simulink model "BRAM_STN_32bit"  (R2021a)
settings: Solver=VariableStepAuto  StartTime=0.0  StopTime=7500.0  RelTol=1e-3
values from neighbouring files (symbols this model uses):
  F_bit = 27    [main.m]
undefined symbols (not defined in the file or in its folder): S, vsva2197, xcvc1902
libraries: xbsIndex_r4 x99, ModelComposer x25, simulink x1
settings Model: Creator=maruf  LastModifiedBy=maruf

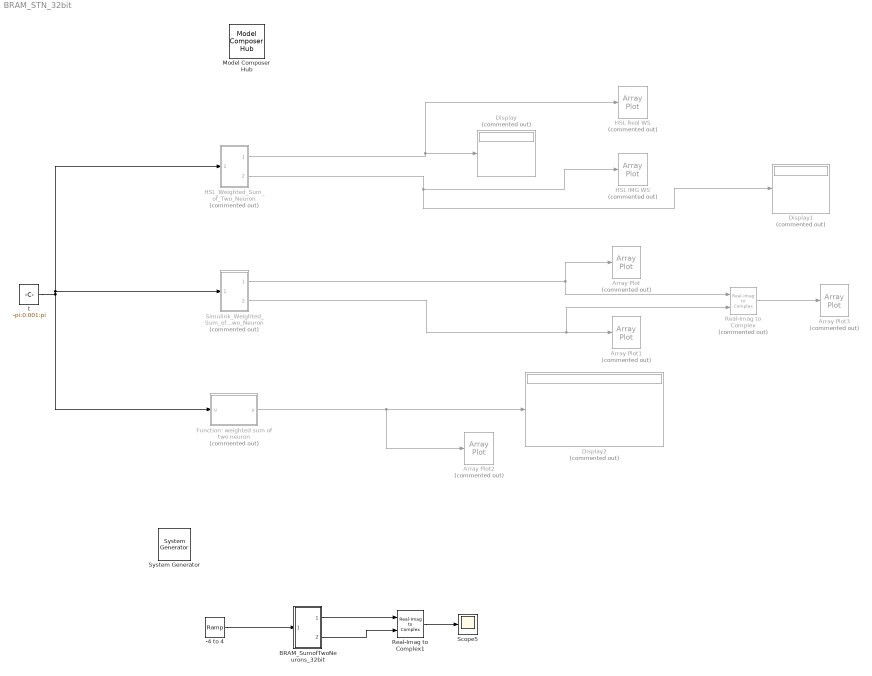
== system BRAM_STN_32bit ==
  " System Generator" : xbsIndex_r4/ System Generator  Tag=genX  xilinxfamily=zynq  part=xc7z020  speed=-1  package=clg484  synthesis_tool=Vivado  clock_wrapper=Clock Enables  directory=E:/FPGAProject/01102022/FPGAResearch/5_Final_Submission/Simulink/BRAM_LT_Based/BRAM32bit/gen_withRegister  proj_type=Vivado  Synth_file=Vivado Synthesis Defaults  Impl_file=Vivado Implementation Defaults  testbench=off  simulink_period=1  sysclk_period=100  dcm_input_clock_period=10  incr_netlist=off  trim_vbits=Everywhere in SubSystem  dbl_ovrd=According to Block Masks  core_generation=According to Block Masks  run_coregen=off  deprecated_control=off  eval_field=0  block_type=sysgen
  -4 to 4 : simulink/Sources/Ramp  slope=1/1000  start=0  InitialOutput=-4
  Array Plot : ArrayPlot  Commented=on  WindowPosition=[5.000000,516.000000,510.000000,316.000000,]  YLimits=[-0.9622504313624441,0.9622504139961428]  DefaultConfigurationName=dsp.scopes.ArrayPlotBlockSpecification
  Array Plot1 : ArrayPlot  Commented=on  WindowPosition=[-2.000000,147.000000,512.000000,337.000000,]  YLimits=[-1.2499999481465376,1.24999953331884]  DefaultConfigurationName=dsp.scopes.ArrayPlotBlockSpecification
  Array Plot2 : ArrayPlot  Commented=on  WindowPosition=[2.000000,179.000000,518.000000,354.000000,]  YLimits=[-1.249996371900796,1.2499673471071675]  ShowLegend=on  DefaultConfigurationName=dsp.scopes.ArrayPlotBlockSpecification
  Array Plot3 : ArrayPlot  Commented=on  WindowPosition=[525.000000,102.000000,526.000000,333.000000,]  YLimits=[-1.249993408699066,1.2499406782915958]  ShowLegend=on  DefaultConfigurationName=dsp.scopes.ArrayPlotBlockSpecification
  BRAM_SumofTwoNeurons_32bit : Subsystem
  Display : Display  Commented=on
  Display1 : Display  Commented=on
  Display2 : Display  Commented=on
  Function: weighted sum of two neuron : MATLAB Function  Commented=on  TreatAsAtomicUnit=on
  HSL IMG WS : ArrayPlot  Commented=on  WindowPosition=[651.000000,15.000000,537.000000,382.000000,]  YLimits=[-1.2499999481465376,1.24999953331884]  DefaultConfigurationName=dsp.scopes.ArrayPlotBlockSpecification
  HSL Real WS : ArrayPlot  Commented=on  WindowPosition=[999.000000,483.000000,539.000000,349.000000,]  YLimits=[-0.9622504313624441,0.9622504139961428]  DefaultConfigurationName=dsp.scopes.ArrayPlotBlockSpecification
  HSL_Weighted_Sum_of_Two_Neuron : Subsystem  Commented=on
  Model Composer Hub : ModelComposer/Model Composer Hub  CodeGeneration=off  SubsystemName=HSL_Weighted_Sum_of_Two_Neuron  TargetDirectory=E:/FPGAProject/01102022/FPGAResearch/25102022_MC/twoNeuron/simulink/code  ExportType=System Generator  IpVendor=xilinx.com  IpLibrary=hls  IpVersion=1.0  IpHWLanguage=Verilog  AieCompilerOptions={}  CreateTestbench=off  TestbenchStackSize=10  RunAieSim=off  AieSimTimeout=50000  RunAieSimProfiling=off  LaunchVitisAnalyzer=off  PlotOutput=off  RunX86Sim=off  X86SimTimeout=10  PlatformType=Not Specified  ProjDevice=xcvc1902-vsva2197-2MP-e-S  ProjDevicePart=xcvc1902-vsva2197-2MP-e-S  SamplePeriod=-1  ClockFrequency=200  DataPathParallelism=1
  Real-Imag to Complex : ModelComposer/Real-Imag to Complex  Commented=on  Input=Real and imag  ConstantPart=0
  Real-Imag to Complex1 : ModelComposer/Real-Imag to Complex  Input=Real and imag  ConstantPart=0
  Scope5 : Scope
  Simulink_Weighted_Sum_of_Two_Neuron : Subsystem  Commented=on
  t : Constant  Value=-pi:0.001:pi
  wires:
  t/1 -> Simulink_Weighted_Sum_of_Two_Neuron/1(In1), HSL_Weighted_Sum_of_Two_Neuron/1(In1), Function: weighted sum of two neuron/1(u)
  Function: weighted sum of two neuron/1(y) -> Array Plot2/1, Display2/1
  Simulink_Weighted_Sum_of_Two_Neuron/1(Out1) -> Array Plot/1, Real-Imag to Complex/1
  Simulink_Weighted_Sum_of_Two_Neuron/2(Out2) -> Real-Imag to Complex/2, Array Plot1/1
  HSL_Weighted_Sum_of_Two_Neuron/1(Out1) -> HSL Real WS/1, Display/1
  HSL_Weighted_Sum_of_Two_Neuron/2(Out2) -> Display1/1, HSL IMG WS/1
  Real-Imag to Complex/1 -> Array Plot3/1
  Real-Imag to Complex1/1 -> Scope5/1
  -4 to 4/1 -> BRAM_SumofTwoNeurons_32bit/1(Input)
  BRAM_SumofTwoNeurons_32bit/1(Out1) -> Real-Imag to Complex1/1
  BRAM_SumofTwoNeurons_32bit/2(Out2) -> Real-Imag to Complex1/2

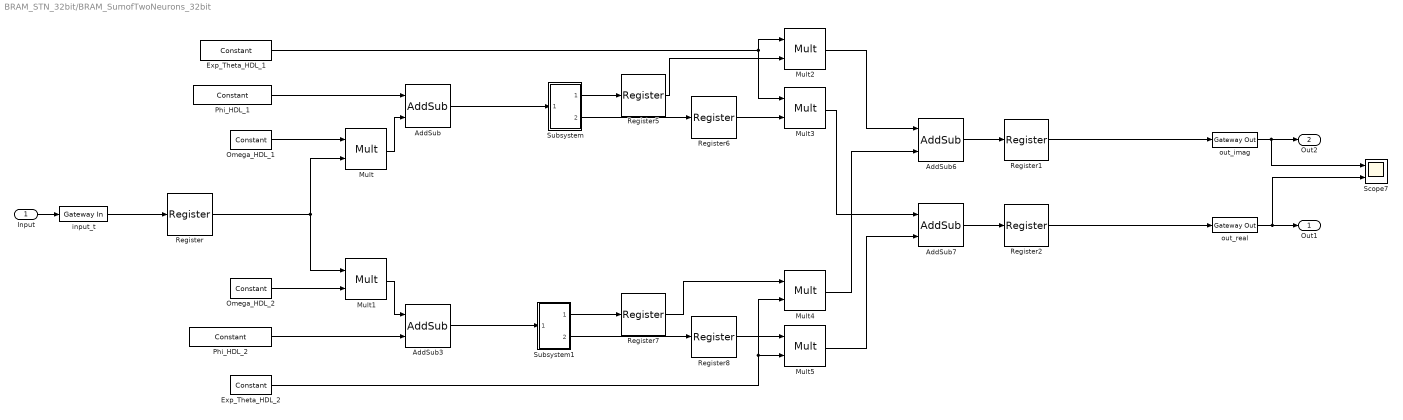
== system BRAM_STN_32bit/BRAM_SumofTwoNeurons_32bit ==
  Input : Inport
  AddSub{,3,6..7} (4 alike) : xbsIndex_r4/AddSub  mode=Addition  use_carryin=off  use_carryout=off  en=off  latency=1  precision=User Defined  arith_type="Signed  (2's comp)"  n_bits=N_bit  bin_pt=F_bit  quantization=Truncate  overflow=Wrap  use_behavioral_HDL=off  hw_selection=Fabric  pipelined=off  dbl_ovrd=off  block_type=addsub
  Exp_Theta_HDL_1 : xbsIndex_r4/Constant  const=2  gui_display_data_type=Fixed-point  arith_type=Signed (2's comp)  n_bits=N_bit  bin_pt=F_bit  preci_type=Single  exp_width=8  frac_width=24  explicit_period=on  period=1  equ=P=C  opselect=C  inp2=PCIN>>17  opr=+  inp1=P  carry=CIN  dbl_ovrd=off  block_type=constant
  Exp_Theta_HDL_2 : xbsIndex_r4/Constant  const=2  gui_display_data_type=Fixed-point  arith_type=Signed (2's comp)  n_bits=N_bit  bin_pt=F_bit  preci_type=Single  exp_width=8  frac_width=24  explicit_period=on  period=1  equ=P=C  opselect=C  inp2=PCIN>>17  opr=+  inp1=P  carry=CIN  dbl_ovrd=off  block_type=constant
  Mult{,1..5} (6 alike) : xbsIndex_r4/Mult  precision=User Defined  arith_type="Signed  (2's comp)"  n_bits=N_bit  bin_pt=F_bit  quantization=Truncate  overflow=Wrap  en=off  latency=3  use_behavioral_HDL=off  opt=Speed  use_embedded=on  optimum_pipeline=off  pipeline=on  dbl_ovrd=off  use_rpm=on  placement_style=Triangular  block_type=mult
  Omega_HDL_1 : xbsIndex_r4/Constant  const=1  gui_display_data_type=Fixed-point  arith_type=Signed (2's comp)  n_bits=N_bit  bin_pt=F_bit  preci_type=Single  exp_width=8  frac_width=24  explicit_period=on  period=1  equ=P=C  opselect=C  inp2=PCIN>>17  opr=+  inp1=P  carry=CIN  dbl_ovrd=off  block_type=constant
  Omega_HDL_2 : xbsIndex_r4/Constant  const=2  gui_display_data_type=Fixed-point  arith_type=Signed (2's comp)  n_bits=N_bit  bin_pt=F_bit  preci_type=Single  exp_width=8  frac_width=24  explicit_period=on  period=1  equ=P=C  opselect=C  inp2=PCIN>>17  opr=+  inp1=P  carry=CIN  dbl_ovrd=off  block_type=constant
  Phi_HDL_1 : xbsIndex_r4/Constant  const=3.14/2  gui_display_data_type=Fixed-point  arith_type=Signed (2's comp)  n_bits=N_bit  bin_pt=F_bit  preci_type=Single  exp_width=8  frac_width=24  explicit_period=on  period=1  equ=P=C  opselect=C  inp2=PCIN>>17  opr=+  inp1=P  carry=CIN  dbl_ovrd=off  block_type=constant
  Phi_HDL_2 : xbsIndex_r4/Constant  const=3.14/2  gui_display_data_type=Fixed-point  arith_type=Signed (2's comp)  n_bits=N_bit  bin_pt=F_bit  preci_type=Single  exp_width=8  frac_width=24  explicit_period=on  period=1  equ=P=C  opselect=C  inp2=PCIN>>17  opr=+  inp1=P  carry=CIN  dbl_ovrd=off  block_type=constant
  Register{,1..2,5..8} (7 alike) : xbsIndex_r4/Register  init=0  rst=off  en=off  dbl_ovrd=off  block_type=register
  Scope7 : Scope  NumInputPorts=2
  Subsystem : Subsystem
  Subsystem1 : Subsystem
  input_t : xbsIndex_r4/Gateway In  gui_display_data_type=Fixed-point  arith_type="Signed  (2's comp)"  n_bits=N_bit  bin_pt=F_bit  preci_type=Single  exp_width=8  frac_width=24  rows=1  columns=1  quantization=Truncate  overflow=Wrap  period=1  UseAsADC=off  ADCChannel='1'  interface=None  automatic_assignment=on  address_offset=hex2dec('00')  intf_name=''  intf_description=''  default_value=0  timing_constraint=None  locs_specified=off  LOCs={}  io_standard={}  inherit_from_input=off  hdl_port=on  dbl_ovrd=off  block_type=gatewayin
  out_imag : xbsIndex_r4/Gateway Out  inherit_from_input=off  hdl_port=on  rows=1  columns=1  UseAsDAC=off  DACChannel='1'  interface=None  automatic_assignment=on  address_offset=hex2dec('00')  intf_name=''  intf_description=''  timing_constraint=None  locs_specified=off  LOCs={}  io_standard={}  block_type=gatewayout
  out_real : xbsIndex_r4/Gateway Out  inherit_from_input=off  hdl_port=on  rows=1  columns=1  UseAsDAC=off  DACChannel='1'  interface=None  automatic_assignment=on  address_offset=hex2dec('00')  intf_name=''  intf_description=''  timing_constraint=None  locs_specified=off  LOCs={}  io_standard={}  block_type=gatewayout
  Out1 : Outport
  Out2 : Outport  Port=2
  wires:
  AddSub/1 -> Subsystem/1(In1)
  Phi_HDL_1/1 -> AddSub/1
  Mult/1 -> AddSub/2
  Omega_HDL_1/1 -> Mult/1
  Exp_Theta_HDL_1/1 -> Mult2/1, Mult3/1
  Omega_HDL_2/1 -> Mult1/2
  Mult1/1 -> AddSub3/1
  Phi_HDL_2/1 -> AddSub3/2
  Exp_Theta_HDL_2/1 -> Mult5/2, Mult4/2
  Mult2/1 -> AddSub6/1
  Mult4/1 -> AddSub6/2
  Mult3/1 -> AddSub7/1
  Mult5/1 -> AddSub7/2
  out_imag/1 -> Out2/1, Scope7/1
  AddSub7/1 -> Register2/1
  out_real/1 -> Scope7/2, Out1/1
  Input/1 -> input_t/1
  input_t/1 -> Register/1
  AddSub6/1 -> Register1/1
  Subsystem/1(Out1) -> Register5/1
  Subsystem/2(Out2) -> Register6/1
  AddSub3/1 -> Subsystem1/1(In1)
  Subsystem1/2(Out2) -> Register8/1
  Subsystem1/1(Out1) -> Register7/1
  Register/1 -> Mult/2, Mult1/1
  Register1/1 -> out_imag/1
  Register2/1 -> out_real/1
  Register5/1 -> Mult2/2
  Register6/1 -> Mult3/2
  Register7/1 -> Mult4/1
  Register8/1 -> Mult5/1

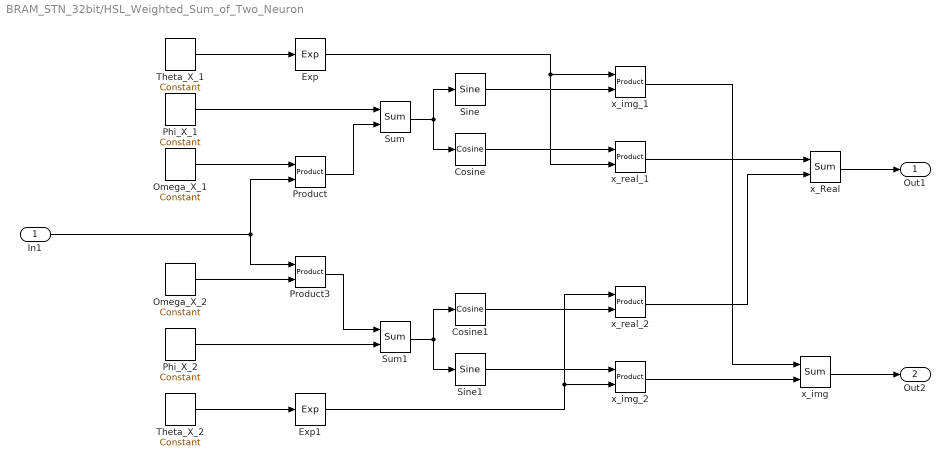
== system BRAM_STN_32bit/HSL_Weighted_Sum_of_Two_Neuron ==
  In1 : Inport
  Cosine : ModelComposer/Cosine
  Cosine1 : ModelComposer/Cosine
  Exp : ModelComposer/Exp
  Exp1 : ModelComposer/Exp
  Omega_X_1 : ModelComposer/Constant  Value=1  VectorParams1D=off  SampleTime=inf  OutDataType=double  TypeExp=''  Signedness=Signed  WordLength=16  FractionalLength=0  RoundingMode=Truncation to minus infinity  OverflowMode=Wrap around
  Omega_X_2 : ModelComposer/Constant  Value=3  SampleTime=inf  OutDataType=double  TypeExp=''  Signedness=Signed  WordLength=16  FractionalLength=0  RoundingMode=Truncation to minus infinity  OverflowMode=Wrap around
  Phi_X_1 : ModelComposer/Constant  Value=pi/2  SampleTime=inf  OutDataType=double  TypeExp=''  Signedness=Signed  WordLength=16  FractionalLength=0  RoundingMode=Truncation to minus infinity  OverflowMode=Wrap around
  Phi_X_2 : ModelComposer/Constant  Value=pi/2  SampleTime=inf  OutDataType=double  TypeExp=''  Signedness=Signed  WordLength=16  FractionalLength=0  RoundingMode=Truncation to minus infinity  OverflowMode=Wrap around
  Product : ModelComposer/Product
  Product3 : ModelComposer/Product
  Sine : ModelComposer/Sine
  Sine1 : ModelComposer/Sine
  Sum : ModelComposer/Sum
  Sum1 : ModelComposer/Sum
  Theta_X_1 : ModelComposer/Constant  Value=log(0.5)  SampleTime=inf  OutDataType=double  TypeExp=''  Signedness=Signed  WordLength=16  FractionalLength=0  RoundingMode=Truncation to minus infinity  OverflowMode=Wrap around
  Theta_X_2 : ModelComposer/Constant  Value=log(0.5)  SampleTime=inf  OutDataType=double  TypeExp=''  Signedness=Signed  WordLength=16  FractionalLength=0  RoundingMode=Truncation to minus infinity  OverflowMode=Wrap around
  x_Real : ModelComposer/Sum
  x_img : ModelComposer/Sum
  x_img_1 : ModelComposer/Product
  x_img_2 : ModelComposer/Product
  x_real_1 : ModelComposer/Product
  x_real_2 : ModelComposer/Product
  Out1 : Outport
  Out2 : Outport  Port=2
  wires:
  Product/1 -> Sum/2
  Cosine/1 -> x_real_1/1
  Sum/1 -> Sine/1, Cosine/1
  Exp/1 -> x_real_1/2, x_img_1/1
  Sine/1 -> x_img_1/2
  In1/1 -> Product/2, Product3/1
  Phi_X_1/1 -> Sum/1
  Omega_X_1/1 -> Product/1
  Omega_X_2/1 -> Product3/2
  Phi_X_2/1 -> Sum1/2
  Product3/1 -> Sum1/1
  Sum1/1 -> Cosine1/1, Sine1/1
  Theta_X_2/1 -> Exp1/1
  Exp1/1 -> x_real_2/1, x_img_2/2
  Sine1/1 -> x_img_2/1
  Cosine1/1 -> x_real_2/2
  x_img/1 -> Out2/1
  x_Real/1 -> Out1/1
  x_real_2/1 -> x_Real/2
  x_real_1/1 -> x_Real/1
  x_img_2/1 -> x_img/2
  x_img_1/1 -> x_img/1
  Theta_X_1/1 -> Exp/1

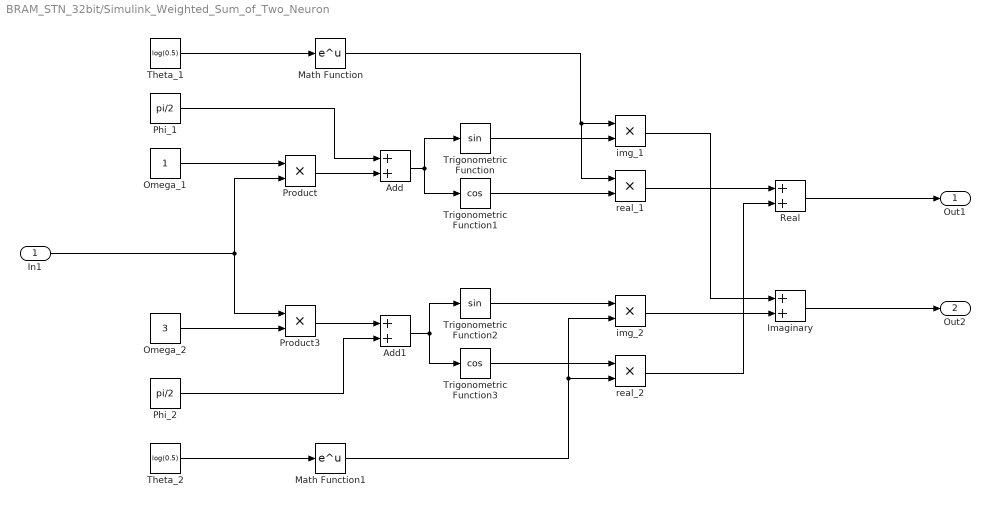
== system BRAM_STN_32bit/Simulink_Weighted_Sum_of_Two_Neuron ==
  In1 : Inport
  Add : Sum
  Add1 : Sum
  Imaginary : Sum
  Math Function : Math  SaturateOnIntegerOverflow=on
  Math Function1 : Math  SaturateOnIntegerOverflow=on
  Omega_1 : Constant
  Omega_2 : Constant  Value=3
  Phi_1 : Constant  Value=pi/2
  Phi_2 : Constant  Value=pi/2
  Product : Product
  Product3 : Product
  Real : Sum
  Theta_1 : Constant  Value=log(0.5)
  Theta_2 : Constant  Value=log(0.5)
  Trigonometric Function : Trigonometry
  Trigonometric Function1 : Trigonometry  Operator=cos
  Trigonometric Function2 : Trigonometry
  Trigonometric Function3 : Trigonometry  Operator=cos
  img_1 : Product
  img_2 : Product
  real_1 : Product
  real_2 : Product
  Out1 : Outport
  Out2 : Outport  Port=2
  wires:
  Theta_2/1 -> Math Function1/1
  Trigonometric Function1/1 -> real_1/2
  real_1/1 -> Real/1
  real_2/1 -> Real/2
  Add/1 -> Trigonometric Function1/1, Trigonometric Function/1
  Omega_1/1 -> Product/1
  Trigonometric Function3/1 -> real_2/1
  Omega_2/1 -> Product3/2
  img_2/1 -> Imaginary/2
  Math Function/1 -> real_1/1, img_1/1
  Trigonometric Function2/1 -> img_2/1
  Theta_1/1 -> Math Function/1
  In1/1 -> Product/2, Product3/1
  Product3/1 -> Add1/1
  Product/1 -> Add/2
  img_1/1 -> Imaginary/1
  Trigonometric Function/1 -> img_1/2
  Math Function1/1 -> img_2/2, real_2/2
  Phi_1/1 -> Add/1
  Add1/1 -> Trigonometric Function2/1, Trigonometric Function3/1
  Real/1 -> Out1/1
  Phi_2/1 -> Add1/2
  Imaginary/1 -> Out2/1

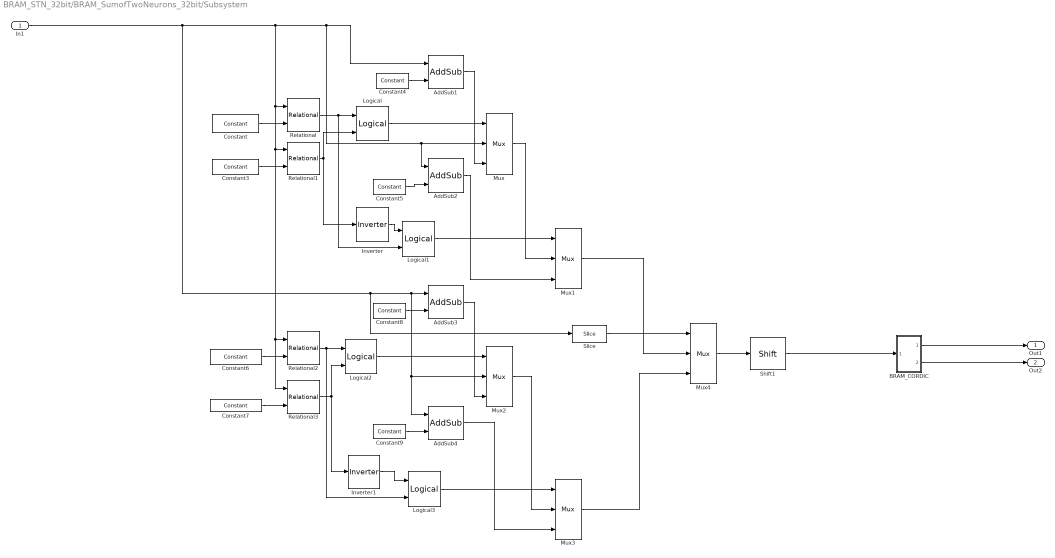
== system BRAM_STN_32bit/BRAM_SumofTwoNeurons_32bit/Subsystem ==
  In1 : Inport
  AddSub1 : xbsIndex_r4/AddSub  mode=Subtraction  use_carryin=off  use_carryout=off  en=off  latency=1  precision=User Defined  arith_type="Signed  (2's comp)"  n_bits=N_bit  bin_pt=F_bit  quantization=Truncate  overflow=Wrap  use_behavioral_HDL=off  hw_selection=Fabric  pipelined=off  dbl_ovrd=off  block_type=addsub
  AddSub2 : xbsIndex_r4/AddSub  mode=Subtraction  use_carryin=off  use_carryout=off  en=off  latency=1  precision=User Defined  arith_type="Signed  (2's comp)"  n_bits=N_bit  bin_pt=F_bit  quantization=Truncate  overflow=Wrap  use_behavioral_HDL=off  hw_selection=Fabric  pipelined=off  dbl_ovrd=off  block_type=addsub
  AddSub3 : xbsIndex_r4/AddSub  mode=Addition  use_carryin=off  use_carryout=off  en=off  latency=1  precision=User Defined  arith_type="Signed  (2's comp)"  n_bits=N_bit  bin_pt=F_bit  quantization=Truncate  overflow=Wrap  use_behavioral_HDL=off  hw_selection=Fabric  pipelined=off  dbl_ovrd=off  block_type=addsub
  AddSub4 : xbsIndex_r4/AddSub  mode=Addition  use_carryin=off  use_carryout=off  en=off  latency=1  precision=User Defined  arith_type="Signed  (2's comp)"  n_bits=N_bit  bin_pt=F_bit  quantization=Truncate  overflow=Wrap  use_behavioral_HDL=off  hw_selection=Fabric  pipelined=off  dbl_ovrd=off  block_type=addsub
  BRAM_CORDIC : Subsystem
  Constant : xbsIndex_r4/Constant  const=3.14  gui_display_data_type=Fixed-point  arith_type=Signed (2's comp)  n_bits=N_bit  bin_pt=F_bit  preci_type=Single  exp_width=8  frac_width=24  explicit_period=on  period=1  equ=P=C  opselect=C  inp2=PCIN>>17  opr=+  inp1=P  carry=CIN  dbl_ovrd=off  block_type=constant
  Constant3 : xbsIndex_r4/Constant  const=9.42  gui_display_data_type=Fixed-point  arith_type=Signed (2's comp)  n_bits=N_bit  bin_pt=F_bit  preci_type=Single  exp_width=8  frac_width=24  explicit_period=on  period=1  equ=P=C  opselect=C  inp2=PCIN>>17  opr=+  inp1=P  carry=CIN  dbl_ovrd=off  block_type=constant
  Constant4 : xbsIndex_r4/Constant  const=6.28  gui_display_data_type=Fixed-point  arith_type=Signed (2's comp)  n_bits=N_bit  bin_pt=F_bit  preci_type=Single  exp_width=8  frac_width=24  explicit_period=on  period=1  equ=P=C  opselect=C  inp2=PCIN>>17  opr=+  inp1=P  carry=CIN  dbl_ovrd=off  block_type=constant
  Constant5 : xbsIndex_r4/Constant  const=12.56  gui_display_data_type=Fixed-point  arith_type=Signed (2's comp)  n_bits=N_bit  bin_pt=F_bit  preci_type=Single  exp_width=8  frac_width=24  explicit_period=on  period=1  equ=P=C  opselect=C  inp2=PCIN>>17  opr=+  inp1=P  carry=CIN  dbl_ovrd=off  block_type=constant
  Constant6 : xbsIndex_r4/Constant  const=-3.14  gui_display_data_type=Fixed-point  arith_type=Signed (2's comp)  n_bits=N_bit  bin_pt=F_bit  preci_type=Single  exp_width=8  frac_width=24  explicit_period=on  period=1  equ=P=C  opselect=C  inp2=PCIN>>17  opr=+  inp1=P  carry=CIN  dbl_ovrd=off  block_type=constant
  Constant7 : xbsIndex_r4/Constant  const=-9.42  gui_display_data_type=Fixed-point  arith_type=Signed (2's comp)  n_bits=N_bit  bin_pt=F_bit  preci_type=Single  exp_width=8  frac_width=24  explicit_period=on  period=1  equ=P=C  opselect=C  inp2=PCIN>>17  opr=+  inp1=P  carry=CIN  dbl_ovrd=off  block_type=constant
  Constant8 : xbsIndex_r4/Constant  const=6.28  gui_display_data_type=Fixed-point  arith_type=Signed (2's comp)  n_bits=N_bit  bin_pt=F_bit  preci_type=Single  exp_width=8  frac_width=24  explicit_period=on  period=1  equ=P=C  opselect=C  inp2=PCIN>>17  opr=+  inp1=P  carry=CIN  dbl_ovrd=off  block_type=constant
  Constant9 : xbsIndex_r4/Constant  const=12.56  gui_display_data_type=Fixed-point  arith_type=Signed (2's comp)  n_bits=N_bit  bin_pt=F_bit  preci_type=Single  exp_width=8  frac_width=24  explicit_period=on  period=1  equ=P=C  opselect=C  inp2=PCIN>>17  opr=+  inp1=P  carry=CIN  dbl_ovrd=off  block_type=constant
  Inverter : xbsIndex_r4/Inverter  en=off  latency=1  dbl_ovrd=off  block_type=inv
  Inverter1 : xbsIndex_r4/Inverter  en=off  latency=1  dbl_ovrd=off  block_type=inv
  Logical{,1..3} (4 alike) : xbsIndex_r4/Logical  logical_function=AND  inputs=2  en=off  latency=1  precision=Full  arith_type=Unsigned  n_bits=16  bin_pt=0  align_bp=on  dbl_ovrd=off  block_type=logical
  Mux{,1..4} (5 alike) : xbsIndex_r4/Mux  inputs=2  en=off  latency=1  precision=Full  arith_type=Unsigned  n_bits=16  bin_pt=14  quantization=Truncate  overflow=Wrap  dbl_ovrd=off  block_type=mux
  Relational : xbsIndex_r4/Relational  mode=a>b  op_type=Bool  en=off  latency=1  dbl_ovrd=off  block_type=relational
  Relational1 : xbsIndex_r4/Relational  mode=a<b  op_type=Bool  en=off  latency=1  dbl_ovrd=off  block_type=relational
  Relational2 : xbsIndex_r4/Relational  mode=a<b  op_type=Bool  en=off  latency=1  dbl_ovrd=off  block_type=relational
  Relational3 : xbsIndex_r4/Relational  mode=a>b  op_type=Bool  en=off  latency=1  dbl_ovrd=off  block_type=relational
  Shift1 : xbsIndex_r4/Shift  shift_dir=Right  shift_bits=0  en=off  latency=1  precision=User Defined  arith_type="Signed  (2's comp)"  n_bits=N_bit  bin_pt=F_bit+2  quantization=Truncate  overflow=Wrap  dbl_ovrd=off  block_type=shift
  Slice : xbsIndex_r4/Slice  nbits=1  boolean_output=on  mode=Upper Bit Location + Width  bit1=0  base1=MSB of Input  bit0=0  base0=LSB of Input  dbl_ovrd=off  block_type=slice
  Out1 : Outport
  Out2 : Outport  Port=2
  wires:
  Logical3/1 -> Mux3/1
  AddSub2/1 -> Mux1/3
  Mux/1 -> Mux1/2
  Mux3/1 -> Mux4/3
  BRAM_CORDIC/1(Out1) -> Out1/1
  BRAM_CORDIC/2(Out2) -> Out2/1
  Mux2/1 -> Mux3/2
  Constant4/1 -> AddSub1/2
  Mux1/1 -> Mux4/2
  Inverter1/1 -> Logical3/1
  AddSub4/1 -> Mux3/3
  Logical2/1 -> Mux2/1
  AddSub1/1 -> Mux/3
  Inverter/1 -> Logical1/1
  Slice/1 -> Mux4/1
  Constant9/1 -> AddSub4/2
  Mux4/1 -> Shift1/1
  Relational/1 -> Logical/1, Logical1/2
  Constant3/1 -> Relational1/2
  Constant8/1 -> AddSub3/2
  Relational1/1 -> Logical/2, Inverter/1
  Constant6/1 -> Relational2/2
  Constant7/1 -> Relational3/2
  Constant5/1 -> AddSub2/2
  Logical1/1 -> Mux1/1
  Logical/1 -> Mux/1
  In1/1 -> Slice/1, AddSub4/1, Mux2/2, AddSub3/1, Relational3/1, Relational2/1, Relational1/1, Relational/1, AddSub2/1, Mux/2, AddSub1/1
  Relational2/1 -> Logical3/2, Logical2/1
  AddSub3/1 -> Mux2/3
  Relational3/1 -> Inverter1/1, Logical2/2
  Constant/1 -> Relational/2
  Shift1/1 -> BRAM_CORDIC/1(In1)

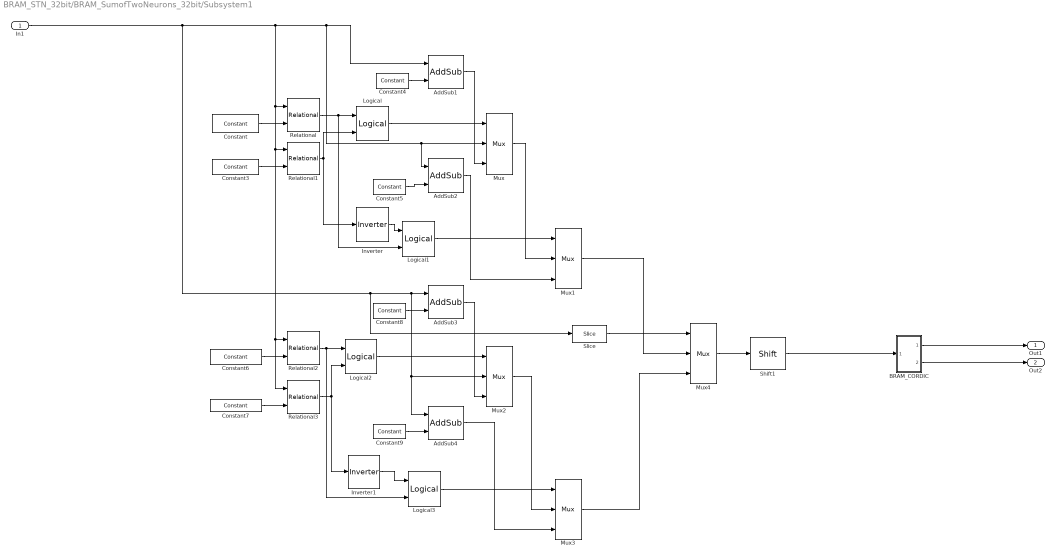
== system BRAM_STN_32bit/BRAM_SumofTwoNeurons_32bit/Subsystem1 ==
  In1 : Inport
  AddSub1 : xbsIndex_r4/AddSub  mode=Subtraction  use_carryin=off  use_carryout=off  en=off  latency=1  precision=User Defined  arith_type="Signed  (2's comp)"  n_bits=N_bit  bin_pt=F_bit  quantization=Truncate  overflow=Wrap  use_behavioral_HDL=off  hw_selection=Fabric  pipelined=off  dbl_ovrd=off  block_type=addsub
  AddSub2 : xbsIndex_r4/AddSub  mode=Subtraction  use_carryin=off  use_carryout=off  en=off  latency=1  precision=User Defined  arith_type="Signed  (2's comp)"  n_bits=N_bit  bin_pt=F_bit  quantization=Truncate  overflow=Wrap  use_behavioral_HDL=off  hw_selection=Fabric  pipelined=off  dbl_ovrd=off  block_type=addsub
  AddSub3 : xbsIndex_r4/AddSub  mode=Addition  use_carryin=off  use_carryout=off  en=off  latency=1  precision=User Defined  arith_type="Signed  (2's comp)"  n_bits=N_bit  bin_pt=F_bit  quantization=Truncate  overflow=Wrap  use_behavioral_HDL=off  hw_selection=Fabric  pipelined=off  dbl_ovrd=off  block_type=addsub
  AddSub4 : xbsIndex_r4/AddSub  mode=Addition  use_carryin=off  use_carryout=off  en=off  latency=1  precision=User Defined  arith_type="Signed  (2's comp)"  n_bits=N_bit  bin_pt=F_bit  quantization=Truncate  overflow=Wrap  use_behavioral_HDL=off  hw_selection=Fabric  pipelined=off  dbl_ovrd=off  block_type=addsub
  BRAM_CORDIC : Subsystem
  Constant : xbsIndex_r4/Constant  const=3.14  gui_display_data_type=Fixed-point  arith_type=Signed (2's comp)  n_bits=N_bit  bin_pt=F_bit  preci_type=Single  exp_width=8  frac_width=24  explicit_period=on  period=1  equ=P=C  opselect=C  inp2=PCIN>>17  opr=+  inp1=P  carry=CIN  dbl_ovrd=off  block_type=constant
  Constant3 : xbsIndex_r4/Constant  const=9.42  gui_display_data_type=Fixed-point  arith_type=Signed (2's comp)  n_bits=N_bit  bin_pt=F_bit  preci_type=Single  exp_width=8  frac_width=24  explicit_period=on  period=1  equ=P=C  opselect=C  inp2=PCIN>>17  opr=+  inp1=P  carry=CIN  dbl_ovrd=off  block_type=constant
  Constant4 : xbsIndex_r4/Constant  const=6.28  gui_display_data_type=Fixed-point  arith_type=Signed (2's comp)  n_bits=N_bit  bin_pt=F_bit  preci_type=Single  exp_width=8  frac_width=24  explicit_period=on  period=1  equ=P=C  opselect=C  inp2=PCIN>>17  opr=+  inp1=P  carry=CIN  dbl_ovrd=off  block_type=constant
  Constant5 : xbsIndex_r4/Constant  const=12.56  gui_display_data_type=Fixed-point  arith_type=Signed (2's comp)  n_bits=N_bit  bin_pt=F_bit  preci_type=Single  exp_width=8  frac_width=24  explicit_period=on  period=1  equ=P=C  opselect=C  inp2=PCIN>>17  opr=+  inp1=P  carry=CIN  dbl_ovrd=off  block_type=constant
  Constant6 : xbsIndex_r4/Constant  const=-3.14  gui_display_data_type=Fixed-point  arith_type=Signed (2's comp)  n_bits=N_bit  bin_pt=F_bit  preci_type=Single  exp_width=8  frac_width=24  explicit_period=on  period=1  equ=P=C  opselect=C  inp2=PCIN>>17  opr=+  inp1=P  carry=CIN  dbl_ovrd=off  block_type=constant
  Constant7 : xbsIndex_r4/Constant  const=-9.42  gui_display_data_type=Fixed-point  arith_type=Signed (2's comp)  n_bits=N_bit  bin_pt=F_bit  preci_type=Single  exp_width=8  frac_width=24  explicit_period=on  period=1  equ=P=C  opselect=C  inp2=PCIN>>17  opr=+  inp1=P  carry=CIN  dbl_ovrd=off  block_type=constant
  Constant8 : xbsIndex_r4/Constant  const=6.28  gui_display_data_type=Fixed-point  arith_type=Signed (2's comp)  n_bits=N_bit  bin_pt=F_bit  preci_type=Single  exp_width=8  frac_width=24  explicit_period=on  period=1  equ=P=C  opselect=C  inp2=PCIN>>17  opr=+  inp1=P  carry=CIN  dbl_ovrd=off  block_type=constant
  Constant9 : xbsIndex_r4/Constant  const=12.56  gui_display_data_type=Fixed-point  arith_type=Signed (2's comp)  n_bits=N_bit  bin_pt=F_bit  preci_type=Single  exp_width=8  frac_width=24  explicit_period=on  period=1  equ=P=C  opselect=C  inp2=PCIN>>17  opr=+  inp1=P  carry=CIN  dbl_ovrd=off  block_type=constant
  Inverter : xbsIndex_r4/Inverter  en=off  latency=1  dbl_ovrd=off  block_type=inv
  Inverter1 : xbsIndex_r4/Inverter  en=off  latency=1  dbl_ovrd=off  block_type=inv
  Logical{,1..3} (4 alike) : xbsIndex_r4/Logical  logical_function=AND  inputs=2  en=off  latency=1  precision=Full  arith_type=Unsigned  n_bits=16  bin_pt=0  align_bp=on  dbl_ovrd=off  block_type=logical
  Mux{,1..4} (5 alike) : xbsIndex_r4/Mux  inputs=2  en=off  latency=1  precision=Full  arith_type=Unsigned  n_bits=16  bin_pt=14  quantization=Truncate  overflow=Wrap  dbl_ovrd=off  block_type=mux
  Relational : xbsIndex_r4/Relational  mode=a>b  op_type=Bool  en=off  latency=1  dbl_ovrd=off  block_type=relational
  Relational1 : xbsIndex_r4/Relational  mode=a<b  op_type=Bool  en=off  latency=1  dbl_ovrd=off  block_type=relational
  Relational2 : xbsIndex_r4/Relational  mode=a<b  op_type=Bool  en=off  latency=1  dbl_ovrd=off  block_type=relational
  Relational3 : xbsIndex_r4/Relational  mode=a>b  op_type=Bool  en=off  latency=1  dbl_ovrd=off  block_type=relational
  Shift1 : xbsIndex_r4/Shift  shift_dir=Right  shift_bits=0  en=off  latency=1  precision=User Defined  arith_type="Signed  (2's comp)"  n_bits=N_bit  bin_pt=F_bit+2  quantization=Truncate  overflow=Wrap  dbl_ovrd=off  block_type=shift
  Slice : xbsIndex_r4/Slice  nbits=1  boolean_output=on  mode=Upper Bit Location + Width  bit1=0  base1=MSB of Input  bit0=0  base0=LSB of Input  dbl_ovrd=off  block_type=slice
  Out1 : Outport
  Out2 : Outport  Port=2
  wires:
  Logical3/1 -> Mux3/1
  AddSub2/1 -> Mux1/3
  Mux/1 -> Mux1/2
  Mux3/1 -> Mux4/3
  BRAM_CORDIC/1(Out1) -> Out1/1
  BRAM_CORDIC/2(Out2) -> Out2/1
  Mux2/1 -> Mux3/2
  Constant4/1 -> AddSub1/2
  Mux1/1 -> Mux4/2
  Inverter1/1 -> Logical3/1
  AddSub4/1 -> Mux3/3
  Logical2/1 -> Mux2/1
  AddSub1/1 -> Mux/3
  Inverter/1 -> Logical1/1
  Slice/1 -> Mux4/1
  Constant9/1 -> AddSub4/2
  Mux4/1 -> Shift1/1
  Relational/1 -> Logical/1, Logical1/2
  Constant3/1 -> Relational1/2
  Constant8/1 -> AddSub3/2
  Relational1/1 -> Logical/2, Inverter/1
  Constant6/1 -> Relational2/2
  Constant7/1 -> Relational3/2
  Constant5/1 -> AddSub2/2
  Logical1/1 -> Mux1/1
  Logical/1 -> Mux/1
  In1/1 -> Slice/1, AddSub4/1, Mux2/2, AddSub3/1, Relational3/1, Relational2/1, Relational1/1, Relational/1, AddSub2/1, Mux/2, AddSub1/1
  Relational2/1 -> Logical3/2, Logical2/1
  AddSub3/1 -> Mux2/3
  Relational3/1 -> Inverter1/1, Logical2/2
  Constant/1 -> Relational/2
  Shift1/1 -> BRAM_CORDIC/1(In1)

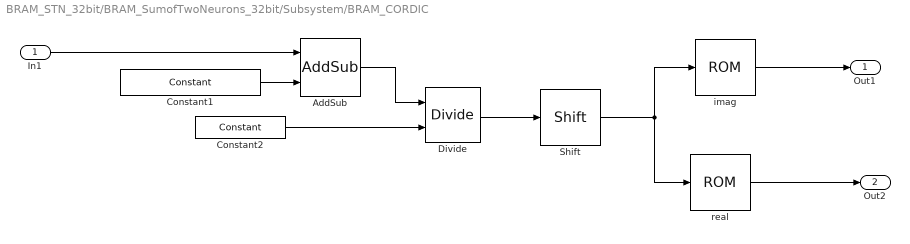
== system BRAM_STN_32bit/BRAM_SumofTwoNeurons_32bit/Subsystem/BRAM_CORDIC ==
  In1 : Inport
  AddSub : xbsIndex_r4/AddSub  mode=Addition  use_carryin=off  use_carryout=off  en=off  latency=1  precision=User Defined  arith_type="Signed  (2's comp)"  n_bits=N_bit  bin_pt=F_bit+1  quantization=Truncate  overflow=Wrap  use_behavioral_HDL=off  hw_selection=Fabric  pipelined=off  dbl_ovrd=off  block_type=addsub
  Constant1 : xbsIndex_r4/Constant  const=3.14  gui_display_data_type=Fixed-point  arith_type=Signed (2's comp)  n_bits=N_bit  bin_pt=F_bit+2  preci_type=Single  exp_width=8  frac_width=24  explicit_period=on  period=1  equ=P=C  opselect=C  inp2=PCIN>>17  opr=+  inp1=P  carry=CIN  dbl_ovrd=off  block_type=constant
  Constant2 : xbsIndex_r4/Constant  const=6.28/629  gui_display_data_type=Fixed-point  arith_type=Signed (2's comp)  n_bits=N_bit  bin_pt=F_bit+2  preci_type=Single  exp_width=8  frac_width=24  explicit_period=on  period=1  equ=P=C  opselect=C  inp2=PCIN>>17  opr=+  inp1=P  carry=CIN  dbl_ovrd=off  block_type=constant
  Divide : xbsIndex_r4/Divide  flow_control=NonBlocking  axi_optimize_goal=Resources  algorithm_type=Radix2  infoedit1=Specify output fraction-width for Fixed-point division.  fractional_width=2  infoedit2=Specify latency for Floating-point division.  latency=1  rate=1  has_a_tlast=off  has_a_tuser=off  has_b_tlast=off  has_b_tuser=off  en=off  has_result_tready=off  result_tlast_behv=Pass_A_TLAST  has_underflow=off  has_overflow=off  has_invalid_op=off  has_divide_by_zero=off  fpo_op_type=mergeddivide  block_type=divide
      settings: infoedit=Blocking: Wait for data on all inputs, allow back-pressure.<br>NonBlocking: operate every cycle in which all inputs are valid, no back-pressure.
  Shift : xbsIndex_r4/Shift  shift_dir=Left  shift_bits=0  en=off  latency=1  precision=User Defined  arith_type=Unsigned  n_bits=10  bin_pt=0  quantization=Truncate  overflow=Wrap  dbl_ovrd=off  block_type=shift
  imag : xbsIndex_r4/ROM  depth=629  initVector=sin(-3.14:0.01:3.14)  distributed_mem=Block RAM  rst=off  init_reg=0  en=off  latency=1  gui_display_data_type=Fixed-point  arith_type="Signed  (2's comp)"  n_bits=N_bit  bin_pt=F_bit+3  preci_type=Single  exp_width=8  frac_width=24  optimize=Area  use_rpm=on  dbl_ovrd=off  simulation_type=fast_sim  block_type=sprom
  real : xbsIndex_r4/ROM  depth=629  initVector=cos(-3.14:0.01:3.14)  distributed_mem=Block RAM  rst=off  init_reg=0  en=off  latency=1  gui_display_data_type=Fixed-point  arith_type="Signed  (2's comp)"  n_bits=N_bit  bin_pt=F_bit+3  preci_type=Single  exp_width=8  frac_width=24  optimize=Area  use_rpm=on  dbl_ovrd=off  simulation_type=fast_sim  block_type=sprom
  Out1 : Outport
  Out2 : Outport  Port=2
  wires:
  Shift/1 -> imag/1, real/1
  Constant1/1 -> AddSub/2
  In1/1 -> AddSub/1
  Constant2/1 -> Divide/2
  Divide/1 -> Shift/1
  AddSub/1 -> Divide/1
  imag/1 -> Out1/1
  real/1 -> Out2/1

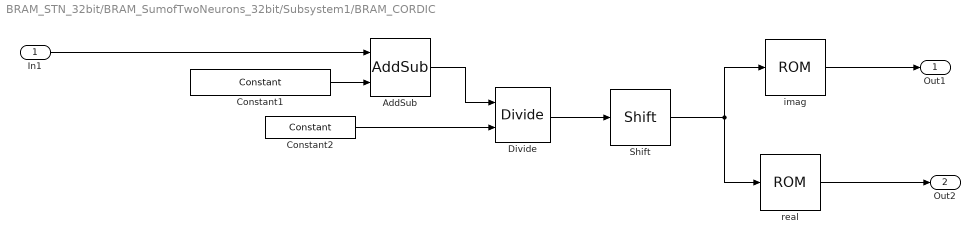
== system BRAM_STN_32bit/BRAM_SumofTwoNeurons_32bit/Subsystem1/BRAM_CORDIC ==
  In1 : Inport
  AddSub : xbsIndex_r4/AddSub  mode=Addition  use_carryin=off  use_carryout=off  en=off  latency=1  precision=User Defined  arith_type="Signed  (2's comp)"  n_bits=N_bit  bin_pt=F_bit+1  quantization=Truncate  overflow=Wrap  use_behavioral_HDL=off  hw_selection=Fabric  pipelined=off  dbl_ovrd=off  block_type=addsub
  Constant1 : xbsIndex_r4/Constant  const=3.14  gui_display_data_type=Fixed-point  arith_type=Signed (2's comp)  n_bits=N_bit  bin_pt=F_bit+2  preci_type=Single  exp_width=8  frac_width=24  explicit_period=on  period=1  equ=P=C  opselect=C  inp2=PCIN>>17  opr=+  inp1=P  carry=CIN  dbl_ovrd=off  block_type=constant
  Constant2 : xbsIndex_r4/Constant  const=6.28/629  gui_display_data_type=Fixed-point  arith_type=Signed (2's comp)  n_bits=N_bit  bin_pt=F_bit+2  preci_type=Single  exp_width=8  frac_width=24  explicit_period=on  period=1  equ=P=C  opselect=C  inp2=PCIN>>17  opr=+  inp1=P  carry=CIN  dbl_ovrd=off  block_type=constant
  Divide : xbsIndex_r4/Divide  flow_control=NonBlocking  axi_optimize_goal=Resources  algorithm_type=Radix2  infoedit1=Specify output fraction-width for Fixed-point division.  fractional_width=2  infoedit2=Specify latency for Floating-point division.  latency=1  rate=1  has_a_tlast=off  has_a_tuser=off  has_b_tlast=off  has_b_tuser=off  en=off  has_result_tready=off  result_tlast_behv=Pass_A_TLAST  has_underflow=off  has_overflow=off  has_invalid_op=off  has_divide_by_zero=off  fpo_op_type=mergeddivide  block_type=divide
      settings: infoedit=Blocking: Wait for data on all inputs, allow back-pressure.<br>NonBlocking: operate every cycle in which all inputs are valid, no back-pressure.
  Shift : xbsIndex_r4/Shift  shift_dir=Left  shift_bits=0  en=off  latency=1  precision=User Defined  arith_type=Unsigned  n_bits=10  bin_pt=0  quantization=Truncate  overflow=Wrap  dbl_ovrd=off  block_type=shift
  imag : xbsIndex_r4/ROM  depth=629  initVector=sin(-3.14:0.01:3.14)  distributed_mem=Block RAM  rst=off  init_reg=0  en=off  latency=1  gui_display_data_type=Fixed-point  arith_type="Signed  (2's comp)"  n_bits=N_bit  bin_pt=F_bit+3  preci_type=Single  exp_width=8  frac_width=24  optimize=Area  use_rpm=on  dbl_ovrd=off  simulation_type=fast_sim  block_type=sprom
  real : xbsIndex_r4/ROM  depth=629  initVector=cos(-3.14:0.01:3.14)  distributed_mem=Block RAM  rst=off  init_reg=0  en=off  latency=1  gui_display_data_type=Fixed-point  arith_type="Signed  (2's comp)"  n_bits=N_bit  bin_pt=F_bit+3  preci_type=Single  exp_width=8  frac_width=24  optimize=Area  use_rpm=on  dbl_ovrd=off  simulation_type=fast_sim  block_type=sprom
  Out1 : Outport
  Out2 : Outport  Port=2
  wires:
  Shift/1 -> imag/1, real/1
  Constant1/1 -> AddSub/2
  In1/1 -> AddSub/1
  Constant2/1 -> Divide/2
  Divide/1 -> Shift/1
  AddSub/1 -> Divide/1
  imag/1 -> Out1/1
  real/1 -> Out2/1

== matlab function BRAM_STN_32bit/Function: weighted sum of two neuron ==
  data: u input; y output
function y = fcn(u)
y = exp((1i*1.*u)+log(0.5))*exp(1i*pi/3)+exp((1i*2.*u)+log(0.5))*exp(1i*pi/3);
